simulink model "inv_rot_pen_sldrt"  (R2024a)
settings: Solver=ode3  StartTime=0.0  StopTime=inf  FixedStep=Ts  RelTol=1e-3
PostLoadFcn:
  | try
  | if isempty(which('ZHAWcbfcn'));
  | callback_fid07124=fopen('ZHAWcbfcn.m','w');
  | [~]=fprintf(callback_fid07124,'%s',get_param([bdroot,'/ Setup SLDRT'],'ClipboardFcn'));
  | [~]=fclose(callback_fid07124);
  | setpref('ZHAW_SLDRT_lib','cb_fcn',which('ZHAWcbfcn'))
  | clear callback_fid07124
  | end
  | catch
  | clear callback_fid07124
  | end
  | Ts=eval(get_param([bdroot,'/ Setup SLDRT'],'Ts'));
InitFcn:
  | Ts=eval(get_param([bdroot,'/ Setup SLDRT'],'Ts'));
values from neighbouring files (symbols this model uses):
  K_oben = lqr(A, B, Q, r)    [inv_rot_pen_ini.m]
  K_unten = lqr(A, B, Q, r)    [inv_rot_pen_ini.m]
  Kp_i = db2mag(8)    [inv_rot_pen_ini.m]
  param = get_parameter()    [inv_rot_pen_ini.m]
  pwm_offset = 0.09    [inv_rot_pen_ini.m]
  Tf = 1 / (2*pi*30)    (= 0.00530516476973)    [inv_rot_pen_ini.m]
  Tn_i = param.L / param.R    [inv_rot_pen_ini.m]
  u_max = 24 * (1 - pwm_offset)    (= 21.84)    [inv_rot_pen_ini.m]
  V_oben = 1 / dc_oben(1)    [inv_rot_pen_ini.m]
  V_unten = 1 / dc_unten(1)    [inv_rot_pen_ini.m]
undefined symbols (not defined in the file or in its folder): National_Instruments, PCIe
libraries: sldrtlib x5, cstblocks x3, simulink x1
(part 2 of 2)

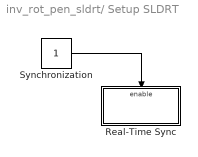
== system inv_rot_pen_sldrt/ Setup SLDRT ==
  Real-Time Sync : Subsystem
  Synchronization : Constant
  wires:
  Synchronization/1 -> Real-Time Sync/Enable

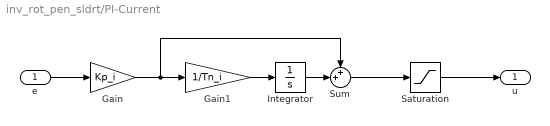
== system inv_rot_pen_sldrt/PI-Current ==
  e : Inport
  Gain : Gain  Gain=Kp_i
  Gain1 : Gain  Gain=1/Tn_i
  Integrator : Integrator  LimitOutput=on  UpperSaturationLimit=u_max  LowerSaturationLimit=-u_max
  Saturation : Saturate  UpperLimit=u_max  LowerLimit=-u_max
  Sum : Sum  Inputs=++|
  u : Outport
  wires:
  Gain1/1 -> Integrator/1
  e/1 -> Gain/1
  Integrator/1 -> Sum/2
  Gain/1 -> Gain1/1, Sum/1
  Sum/1 -> Saturation/1
  Saturation/1 -> u/1

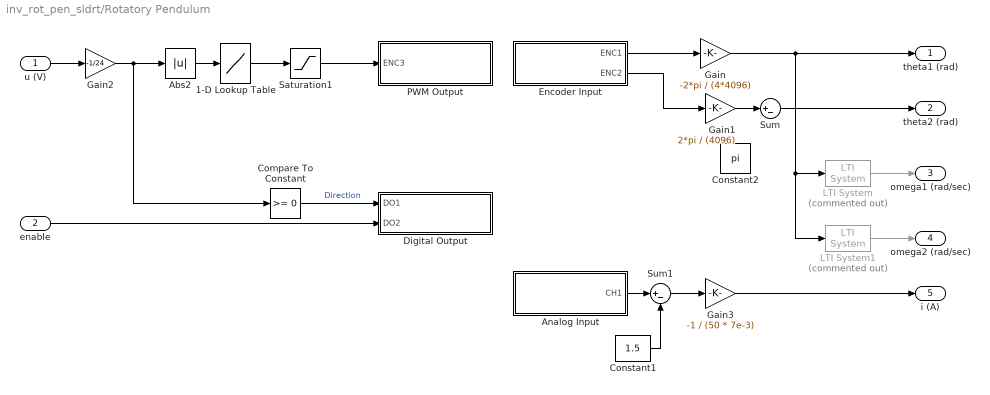
== system inv_rot_pen_sldrt/Rotatory Pendulum ==
  u (V) : Inport
  enable : Inport  Port=2
  1-D Lookup Table : Lookup_n-D  NumberOfTableDimensions=1  BreakpointsForDimension1=[0, 0.0001, 1]  Table=[0, pwm_offset, 1+pwm_offset]  InternalRulePriority=Speed  RndMeth=Simplest
  Abs2 : Abs  SaturateOnIntegerOverflow=off
  Analog Input : Subsystem  mask(NI Analog Input){device=PCIe-6321, connect=Banana Terminal, couple=differential, ch1=on, ch9=off, ch2=off, ch10=off, ch3=off, ch11=off, ch4=off, ch12=off, ch5=off, ch13=off, ch6=off, ch14=off, ch7=off, ch15=off, ch8=off, ch16=off, Ts=Ts}
      mask prompts: device "NI Device Type:"; connect "Connector Box:"; couple "CH Coupling:"; ch1 "CH1-CH9"; ch9 "CH9-GND"; ch2 "CH2-CH10"; ch10 "CH10-GND"; ch3 "CH3-CH11"; ch11 "CH11-GND"; ch4 "CH4-CH12"; ch12 "CH12-GND"; ch5 "CH5-CH13"; ch13 "CH13-GND"; ch6 "CH6-CH14"; ch14 "CH14-GND"; ch7 "CH7-CH15"; ch15 "CH15-GND"; ch8 "CH8-CH16"; ch16 "CH16-GND"; Ts "Sample Time:"
      mask help:
      | AD Converter
      | +/-10V
      mask init:
      | try ch_list = ZHAWcbfcn('get_ch_list'); end
      | try ZHAWcbfcn('BlockUpdate'); end
      settings: AttributesFormatString=%<couple>  OpenFcn=try ZHAWcbfcn('openMask'); end
      settings: CopyFcn=|
      | try
      | ZHAWcbfcn('CopyIOblock')
      | end
      | set_param(gcb,'OpenFcn','try ZHAWcbfcn(''openMask''); end')
      mask TypeOptions device: PCI-6221 | PCI-6259 | PCIe-6259 | PCIe-6321 | PCIe-6363
      mask TypeOptions connect: BNC Terminal | Banana Terminal | Screw Terminal
      mask Callback connect:
      | try ZHAWcbfcn('SetConnectorBox'); end
      | try ZHAWcbfcn('SetChannelCoupling'); end
      mask TypeOptions couple: single ended | differential
      mask Callback couple:
      | try ZHAWcbfcn('SetChannelCoupling'); end
      | try ZHAWcbfcn('SetConnectorBox'); end
      mask DialogControl DescGroupVar Prompt: NI Analog Input (R2024a)
      mask Display: disp('NI\nPCIe-6321')
  Compare To Constant : simulink/Logic and Bit Operations/Compare To Constant  relop=>=  const=0  OutDataTypeStr=boolean
  Constant1 : Constant  Value=1.5
  Constant2 : Constant  Value=pi
  Digital Output : Subsystem  mask(NI Digital Output){device=PCIe-6321, connect=Banana Terminal, ch1=on, ch2=on, ch3=off, ch4=off, ch5=off, ch6=off, ch7=off, ch8=off, Ts=Ts}
      mask prompts: device "NI Device Type:"; connect "Connector Box:"; ch1 "DO1"; ch2 "DO2"; ch3 "DO3"; ch4 "DO4"; ch5 "DO5"; ch6 "DO6"; ch7 "DO7"; ch8 "DO8"; Ts "Sample Time:"
      mask help: Digital output 5V TTL.
      mask init:
      | try ch_list = ZHAWcbfcn('get_ch_list'); end
      | try ZHAWcbfcn('BlockUpdate'); end
      settings: OpenFcn=try ZHAWcbfcn('openMask'); end
      settings: CopyFcn=|
      | try
      | ZHAWcbfcn('CopyIOblock')
      | end
      | set_param(gcb,'OpenFcn','try ZHAWcbfcn(''openMask''); end')
      mask TypeOptions device: PCI-6221 | PCI-6259 | PCIe-6259 | PCIe-6321 | PCIe-6363
      mask Callback device: try ZHAWcbfcn('SetChannelNumber'); end
      mask TypeOptions connect: BNC Terminal | Banana Terminal | Screw Terminal
      mask Callback connect: try ZHAWcbfcn('SetConnectorBox'); end
      mask DialogControl DescGroupVar Prompt: NI Digital Output (R2024a)
      mask Display: disp('NI\nPCIe-6321')
  Encoder Input : Subsystem  mask(NI Encoder Input){device=PCIe-6321, connect=Banana Terminal, reset=off, ch1=on, ch2=on, ch3=off, ch4=off, Ts=Ts}
      mask prompts: device "NI Device Type:"; connect "Connector Box:"; reset "Reset at Index:"; ch1 "ENC1"; ch2 "ENC2"; ch3 "ENC3"; ch4 "ENC4"; Ts "Sample Time:"
      mask help:
      | Quadratur Encoder.
      | X4 Decoding.
      | Output is increments.
      mask init:
      | try ch_list = ZHAWcbfcn('get_ch_list'); end
      | try ZHAWcbfcn('BlockUpdate'); end
      settings: AttributesFormatString=Index Reset: %<reset>  OpenFcn=try ZHAWcbfcn('openMask'); end
      settings: CopyFcn=|
      | try
      | ZHAWcbfcn('CopyIOblock')
      | end
      | set_param(gcb,'OpenFcn','try ZHAWcbfcn(''openMask''); end')
      mask TypeOptions device: PCI-6221 | PCI-6259 | PCIe-6259 | PCIe-6321 | PCIe-6363
      mask Callback device: try ZHAWcbfcn('SetChannelNumber'); end
      mask TypeOptions connect: BNC Terminal | Banana Terminal | Screw Terminal
      mask Callback connect: try ZHAWcbfcn('SetConnectorBox'); end
      mask TypeOptions reset: on | off
      mask Callback reset: try ZHAWcbfcn('SetEncoderReset'); end
      mask DialogControl DescGroupVar Prompt: NI Encoder Input (R2024a)
      mask Display: disp('NI\nPCIe-6321')
  Gain : Gain  Gain=-2*pi / (4*4096)
  Gain1 : Gain  Gain=2*pi / (4096)
  Gain2 : Gain  Gain=-1/24
  Gain3 : Gain  Gain=-1 / (50 * 7e-3)
  LTI System : cstblocks/LTI System  Commented=on  sys=G_diff  IC=[]  PadeOrder=0
  LTI System1 : cstblocks/LTI System  Commented=on  sys=G_diff  IC=[]  PadeOrder=0
  PWM Output : Subsystem  mask(NI PWM Output){device=PCIe-6321, connect=Banana Terminal, mode=PWM, ch1=off, ch2=off, ch3=on, ch4=off, pwm_frequ=20e3, duty=0, Ts_copy=Ts}
      mask prompts: device "NI Device Type:"; connect "Connector Box :"; mode "Output Modus:"; ch1 "ENC1"; ch2 "ENC2"; ch3 "ENC3"; ch4 "ENC4"; pwm_frequ "PWM Frequency [Hz]:"; duty "Duty Cycle [0...1]:"; Ts_copy "Sample Time:"
      mask help:
      | PWM or Frequency output.
      |
      | PWM:
      | The input specifies the duty cycle as a decimal fraction from 0 through 1 inclusive.
      | It determines the amount of time that the output signal value is high (1).
      |
      | Frequency;
      | The input specifies the output frequency in [Hz].
      mask init:
      | try ch_list = ZHAWcbfcn('get_ch_list'); end
      | try ZHAWcbfcn('BlockUpdate'); end
      settings: OpenFcn=try ZHAWcbfcn('openMask'); end
      settings: CopyFcn=|
      | try
      | ZHAWcbfcn('CopyIOblock')
      | end
      | set_param(gcb,'OpenFcn','try ZHAWcbfcn(''openMask''); end')
      mask TypeOptions device: PCI-6221 | PCI-6259 | PCIe-6259 | PCIe-6321 | PCIe-6363
      mask Callback device: try ZHAWcbfcn('SetChannelNumber'); end
      mask TypeOptions connect: BNC Terminal | Banana Terminal | Screw Terminal
      mask Callback connect: try ZHAWcbfcn('SetConnectorBox'); end
      mask TypeOptions mode: PWM | Frequency
      mask DialogControl DescGroupVar Prompt: NI Analog Output (R2024a)
      mask Display: disp('NI\nPCIe-6321')
  Saturation1 : Saturate  UpperLimit=1  LowerLimit=0
  Sum : Sum  Inputs=|+-
  Sum1 : Sum  Inputs=|+-
  theta1 (rad) : Outport
  theta2 (rad) : Outport  Port=2
  omega1 (rad/sec) : Outport  Port=3
  omega2 (rad/sec) : Outport  Port=4
  i (A) : Outport  Port=5
  wires:
  Compare To Constant/1 -> Digital Output/1(DO1)  "Direction"
  Gain/1 -> LTI System1/1, LTI System/1, theta1 (rad)/1
  Encoder Input/1(ENC1) -> Gain/1
  Gain2/1 -> Compare To Constant/1, Abs2/1
  u (V)/1 -> Gain2/1
  enable/1 -> Digital Output/2(DO2)
  Analog Input/1(CH1) -> Sum1/1
  Abs2/1 -> 1-D Lookup Table/1
  1-D Lookup Table/1 -> Saturation1/1
  Saturation1/1 -> PWM Output/1(ENC3)
  Constant1/1 -> Sum1/2
  Sum1/1 -> Gain3/1
  LTI System/1 -> omega1 (rad/sec)/1
  Gain3/1 -> i (A)/1
  Encoder Input/2(ENC2) -> Gain1/1
  Gain1/1 -> Sum/1
  Sum/1 -> theta2 (rad)/1
  LTI System1/1 -> omega2 (rad/sec)/1

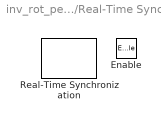
== system inv_rot_pen_sldrt/ Setup SLDRT/Real-Time Sync ==
  Enable : EnablePort
  Real-Time Synchronization : sldrtlib/Real-Time Synchronization  SampleTime=Ts  MaxMissedTicks=inf  ShowMissedTicks=off  YieldWhenWaiting=off

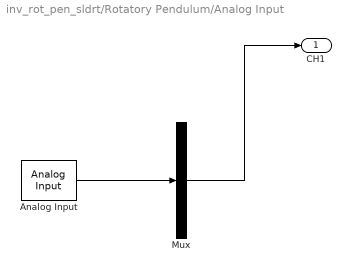
== system inv_rot_pen_sldrt/Rotatory Pendulum/Analog Input ==
  Analog Input : sldrtlib/Analog Input  SampleTime=Ts  MaxMissedTicks=10  ShowMissedTicks=off  YieldWhenWaiting=off  DrvName=National_Instruments/PCIe-6321  DrvAddress=4294967295  DrvOptions="[1  3  0  2  2  3  2]"  Channels=ch_list  RangeMode=1  VoltRange=1  DataType=1
      settings: AttributesFormatString=National Instruments\nPCIe-6321 [auto]
  Mux : Demux  Outputs=1
  CH1 : Outport  VectorParamsAs1DForOutWhenUnconnected=off
  wires:
  Mux/1 -> CH1/1
  Analog Input/1 -> Mux/1

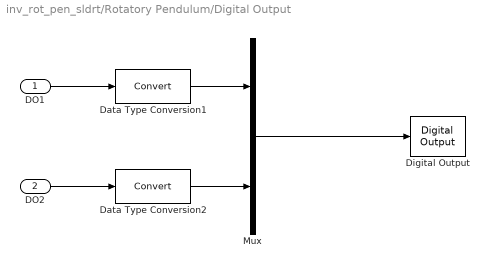
== system inv_rot_pen_sldrt/Rotatory Pendulum/Digital Output ==
  DO1 : Inport
  DO2 : Inport  Port=2
  Data Type Conversion1 : DataTypeConversion  SaturateOnIntegerOverflow=off  RndMeth=Floor
  Data Type Conversion2 : DataTypeConversion  SaturateOnIntegerOverflow=off  RndMeth=Floor
  Digital Output : sldrtlib/Digital Output  SampleTime=Ts  MaxMissedTicks=10  ShowMissedTicks=off  YieldWhenWaiting=off  DrvName=National_Instruments/PCIe-6321  DrvAddress=4294967295  DrvOptions="[1  3  0  2  2  3  2]"  Channels=ch_list  BitMode=1  InitialValue=0  FinalValue=0
      settings: AttributesFormatString=National Instruments\nPCIe-6321 [auto]
  Mux : Mux  Inputs=2
  wires:
  DO1/1 -> Data Type Conversion1/1
  DO2/1 -> Data Type Conversion2/1
  Mux/1 -> Digital Output/1
  Data Type Conversion1/1 -> Mux/1
  Data Type Conversion2/1 -> Mux/2

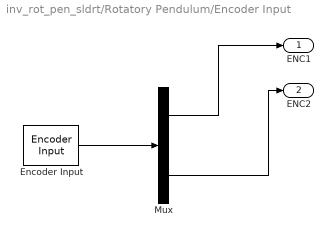
== system inv_rot_pen_sldrt/Rotatory Pendulum/Encoder Input ==
  Encoder Input : sldrtlib/Encoder Input  SampleTime=Ts  MaxMissedTicks=10  ShowMissedTicks=off  YieldWhenWaiting=off  DrvName=National_Instruments/PCIe-6321  DrvAddress=4294967295  DrvOptions="[1  3  0  2  2  3  2]"  Channels=ch_list  QuadMode=3  IndexPulse=1  InputFilter=Inf  DataType=1
      settings: AttributesFormatString=National Instruments\nPCIe-6321 [auto]
  Mux : Demux  Outputs=2
  ENC1 : Outport  VectorParamsAs1DForOutWhenUnconnected=off
  ENC2 : Outport  Port=2
  wires:
  Encoder Input/1 -> Mux/1
  Mux/1 -> ENC1/1
  Mux/2 -> ENC2/1

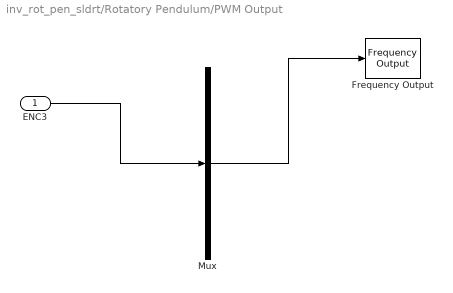
== system inv_rot_pen_sldrt/Rotatory Pendulum/PWM Output ==
  ENC3 : Inport
  Frequency Output : sldrtlib/Frequency Output  SampleTime=Ts  MaxMissedTicks=10  ShowMissedTicks=off  YieldWhenWaiting=off  DrvName=National_Instruments/PCIe-6321  DrvAddress=4294967295  DrvOptions="[1  3  0  2  2  3  2]"  Channels=ch_list  FrequencySource=1  Frequency=20e3  FrequencyFinalValue=20e3  DutySource=2  Duty=0  DutyFinalValue=0
      settings: AttributesFormatString=National Instruments\nPCIe-6321 [auto]
  Mux : Mux  Inputs=1
  wires:
  Mux/1 -> Frequency Output/1
  ENC3/1 -> Mux/1

== matlab function inv_rot_pen_sldrt/Controller ==
  settings: updateMethod=DISCRETE  sampleTime=Ts
  data theta_2 settings: description=(rad)
  data: theta_1 input; theta_2 input; i output size=1; param parameter; k input; switch_angle input; switch_position input; K_oben parameter; K_unten parameter; Ts parameter; Tf parameter; states output; E output; u_acc output; omega1_soll input; V_unten parameter; V_oben parameter
function [i, states, E, u_acc] = fcn(theta_1, theta_2, param, k, switch_angle, switch_position, K_oben, K_unten, Ts, Tf, omega1_soll, V_unten, V_oben)

    % Persistente Variablen für Zustände und Filter
    persistent mode theta_1_offset r_soll
    if isempty(mode)
        mode = 0;  % Start im Modus 0: unten regeln
        theta_1_offset = 0;
        r_soll = 0;
    end

    % Initialisierung für Coder
    i = 0;
    states = zeros(4,1); 
    E = 0;
    u_acc = 0;
    

    % Filterung der Winkelgeschwindigkeit
    [omega_1f, omega_2f] = filter_velocity(theta_1, theta_2, Ts, Tf);

    % Normierter Winkel für obenregelung (theta_2_up = 0 wenn oben)
    theta_2_up = abs(mod(theta_2, 2*pi) - pi);

    % Geschwindigkeitsvorgabe Motor
    r_soll = velocity_control_motor(r_soll, omega1_soll, Ts);

   switch mode
    case 0  % Unten regeln
        theta_2_short = atan2(sin(theta_2), cos(theta_2));
        states = [theta_1-theta_1_offset; theta_2_short; omega_1f; omega_2f];

        if switch_position == 1
            mode = 1;  % Wechsel zu Aufschwingen
        elseif theta_2_up >= 90 * pi / 180
            i = (r_soll*V_unten) - K_unten * states;
            % disp('Regeln unten');
        else
            i = 0;
            theta_1_offset = theta_1;
            r_soll = 0;
            % disp('Abschwingen');
        end

    case 1  % Aufschwingen
        % Energie Berechnung für Aufschwingen
        [i, E, u_acc] = calc_upswing(theta_2, omega_2f, omega_1f, param, k);
        theta_2_short = atan2(sin(theta_2 + pi), cos(theta_2 + pi));
        states = [theta_1; theta_2_short; omega_1f; omega_2f];
        % disp('Aufschwingen');
        if switch_position > 0 && theta_2_up <= switch_angle * pi / 180
            mode = 2;  % Umschalten auf oben regeln
            theta_1_offset = theta_1;
            r_soll = 0;
        end
        if switch_position == 0
            mode = 0;  % Umschalten auf abschwingen / unten regelen
        end

    case 2  % Oben regeln   
        theta_2_short = atan2(sin(theta_2 + pi), cos(theta_2+ pi));
        states = [theta_1-theta_1_offset; theta_2_short; omega_1f; omega_2f];
        i = r_soll * V_oben - K_oben * states;
        % disp('Regeln oben');

        if theta_2_up > switch_angle * pi / 180
            mode = 1; % Umschalten auf Aufschwingen
        end

        if switch_position == 0 
            mode = 0;  % Umschalten auf abschwingen / unten regeln
        end

    case 3 % Geschwindigkeits Überschreitung
           theta_2_short = atan2(sin(theta_2), cos(theta_2));
           states = [theta_1-theta_1_offset; theta_2_short; omega_1f; omega_2f];
           i = 0;

   end

    % Kompensation der Haftreibung
    i = sign(i)*0.0205+i;

    % Begrenzung Motor
    [mode, i] = motor_limit(param, omega_1f, i, mode);
    
end

function [omega_1f, omega_2f] = filter_velocity(theta_1, theta_2, Ts, Tf_sim)
    persistent theta_1_past theta_2_past omega_1f_past omega_2f_past a b
    if isempty(theta_1_past)
        theta_1_past = theta_1;
        theta_2_past = theta_2;
        omega_1f_past = 0;
        omega_2f_past = 0;
        b = 2.0 / (2*Tf_sim + Ts);
        a = (Ts - 2*Tf_sim) / (2*Tf_sim + Ts);
    end

    omega_1f = b * (theta_1 - theta_1_past) - a * omega_1f_past;
    omega_2f = b * (theta_2 - theta_2_past) - a * omega_2f_past;

    theta_1_past = theta_1;
    theta_2_past = theta_2;
    omega_1f_past = omega_1f;
    omega_2f_past = omega_2f;
end

function [i, E, u_acc] = calc_upswing(theta_2, omega_2f, omega_1f, param, k)
    persistent J J_arm Er
    if isempty(J)
        J = param.m2 * param.L2^2 / 12; % Trägheitmoment des Pendels
        J_arm = param.J1zz;
        Er = 2 * param.m2 * param.g * param.l2;
    end

    E = 0.5 * J * omega_2f^2 + param.m2 * -param.g * param.l2 * (cos(theta_2)-1);
    u_acc = k * (E - Er) * sign(omega_2f * cos(theta_2));  % Energie-Regelung
    % u = u_acc * param.m1 * param.L1 * param.Rm / param.kt; % Spannungsberechnung wie bei Quanser
    i = (u_acc / param.L1) * J_arm / param.km - 0.005*omega_1f;
end

function [mode, i] = motor_limit(param, omega_1f, i, mode)
    %Geschwindigkeitsbegrenzung Motor
    if abs(omega_1f) > 35
        mode = 3;
    end
    % Begrenzung auf ±1A
    i = min(max(i, -param.i_max_setpoint), param.i_max_setpoint);
end

function r_soll = velocity_control_motor(r_soll, omega1_soll, Ts)
    % Mindesgestgeschwindigkeit Slider Motor
    if abs(omega1_soll) < 0.15
        omega1_soll = 0;
    end
    % Saturation auf max 1 U/s
    omega1_sat = min(max(omega1_soll, -2*pi), 2*pi);
    r_soll = Ts*(omega1_sat) + r_soll;
end
